simulink library "smartTruckLib"  (R2018b)
settings: Solver=VariableStepAuto  StartTime=0.0  StopTime=10.0  RelTol=1e-3
values from neighbouring files (symbols this model uses):
  actorDest = 0    [modelParams.m]
  initYPos = 0    [modelParams.m]
  laneWidth = laneSpecification.Width    [modelParams.m]
  minOverlapJourney = 200    [modelParams.m]
  platoonFuelSavings = 20    [modelParams.m]
  safeTimeGap = 1.4    [modelParams.m]
  standStillGap = 10    [modelParams.m]
undefined symbols (not defined in the file or in its folder): DiscIntNeverNeededParam, key, setActorTableEntry, tableEntry
libraries: mpcadaslib x1
settings Model: Creator=surongal  LastModifiedBy=surongal
settings DataIOCC: ReturnWorkspaceOutputs=on

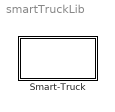
== system smartTruckLib ==
  Smart-Truck : Subsystem  InitFcn=|  mask(Truck){initXPos=100, destXPos=5000, initXVel=10, maxAcceleration=3, maxDeceleration=-6, maxVelocity=30, truckId=1}
      | % To get the offset for the truckId
      | numTrucks = actorCount();
      | truckXPosition(numTrucks) = str2num( get_param(gcb,'initXPos'));
      | truckVelocity(numTrucks) = str2num( get_param(gcb,'initXVel'));
      | % To set the truckId
      | set_param(gcb,'truckId',num2str(numTrucks + truckIdBase));
      | destXPos = get_param(gcb,'destXPos');
      | actorDest(truckIdBase + numTrucks) = str2num(destXPos);
      mask prompts: initXPos "Initial X-position"; destXPos "Destination X-Position"; initXVel "Initial X-velocity"; maxAcceleration "Max acceleration"; maxDeceleration "Max deceleration"; maxVelocity "Max velocity"; truckId "id"
      mask help: This block allows to introduce a smart-truck in the scenario.
      mask Display: image('icons/truck.png');

== system smartTruckLib/Smart-Truck ==
  note: Smart Truck
  Actor-system : Subsystem
  Bus Selector : BusSelector  OutputSignals=ActorID
  Load Initial Pose : MATLAB Function  TreatAsAtomicUnit=on
  Publish to Table : FunctionCaller  FunctionPrototype=setActorTableEntry(key,tableEntry)
  wires:
  Load Initial Pose/1(initTruckPose) -> Actor-system/1(Initial Truck Pose)
  Actor-system/1(Updated Pose) -> Publish to Table/2, Bus Selector/1
  Bus Selector/1 -> Publish to Table/1  "<ActorID>"

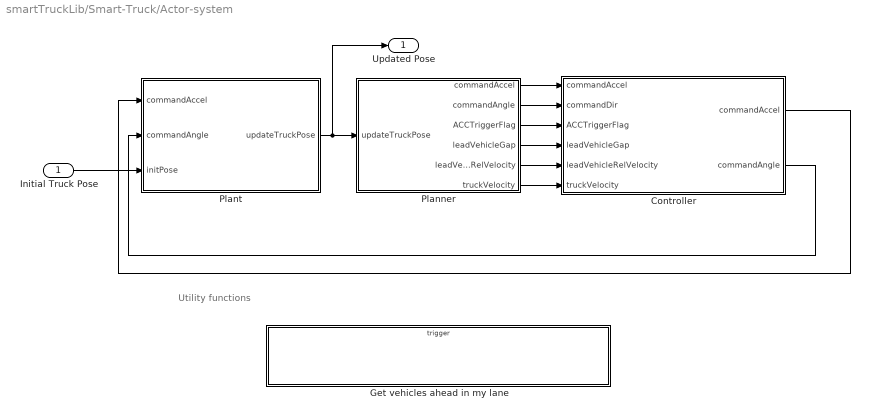
== system smartTruckLib/Smart-Truck/Actor-system ==
  note: Utility functions
  Initial Truck Pose : Inport
  Controller : Subsystem
  Get vehicles ahead in my lane : Subsystem  TreatAsAtomicUnit=on
  Planner : Subsystem
  Plant : Subsystem
  Updated Pose : Outport
  wires:
  Planner/6(truckVelocity) -> Controller/6(" truckVelocity")
  Planner/5(leadVehicleRelVelocity) -> Controller/5(" leadVehicleRelVelocity")
  Planner/4(leadVehicleGap) -> Controller/4(" leadVehicleGap")
  Planner/3(ACCTriggerFlag) -> Controller/3(ACCTriggerFlag)
  Planner/2(commandAngle) -> Controller/2(" commandDir")
  Planner/1(commandAccel) -> Controller/1(" commandAccel")
  Plant/1(updateTruckPose) -> Updated Pose/1, Planner/1(updateTruckPose)
  Controller/1(commandAccel) -> Plant/1(" commandAccel")
  Initial Truck Pose/1 -> Plant/3(initPose)
  Controller/2(commandAngle) -> Plant/2(commandAngle)

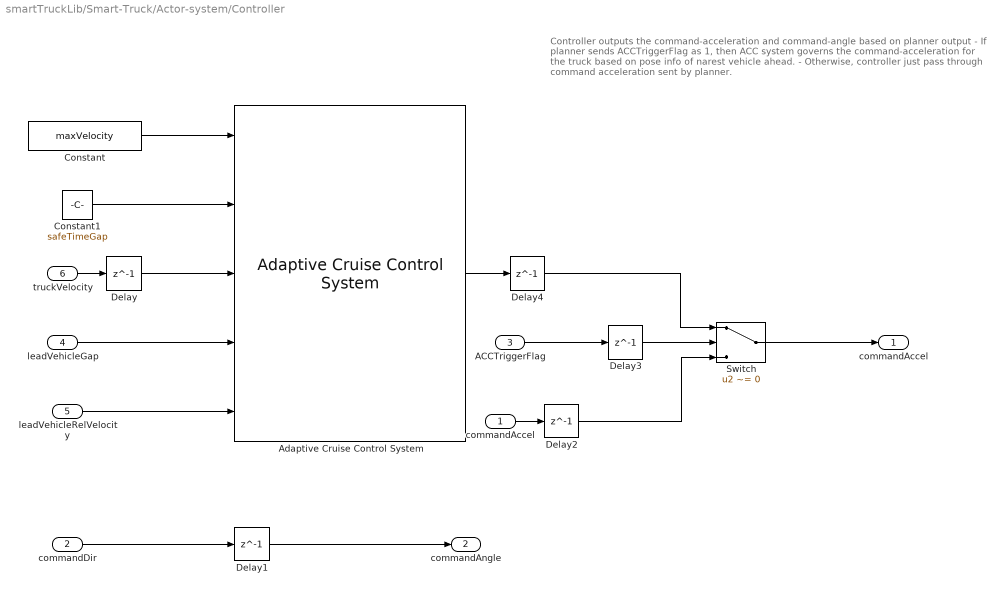
== system smartTruckLib/Smart-Truck/Actor-system/Controller ==
  note: Controller outputs the command-acceleration and command-angle
      | based on planner output
      | - If planner sends ACCTriggerFlag as 1, then ACC system governs the
      |   command-acceleration for the truck based on pose info
      |   of narest vehicle ahead.
      | - Otherwise, controller just pass through command acceleration
      |   sent by planner.
  " commandAccel" : Inport
  " commandDir" : Inport  Port=2
  ACCTriggerFlag : Inport  Port=3
  " leadVehicleGap" : Inport  Port=4
  " leadVehicleRelVelocity" : Inport  Port=5
  " truckVelocity" : Inport  Port=6
  Adaptive Cruise Control System : mpcadaslib/Adaptive Cruise Control System  EgoModel=tf(1,[0.5,1,0])  InitialEgoVelocity=abs(initXVel)  DefaultSpacing=standStillGap  MaxVelocity=maxVelocity  MinAcceleration=maxDeceleration  amin_ext=off  MaxAcceleration=maxAcceleration  amax_ext=off  Ts=0.1  PredictionHorizon=30  ControllerBehavior=0.5  suboptimal=off  maxiter=10  datatypeopt=double  optmode=off  trackmode=off
      settings: SourceProductName=Model Predictive Control Toolbox
  Constant : Constant  Value=maxVelocity  SampleTime=-1
  Constant1 : Constant  Value=safeTimeGap
  Delay{,1..4} (5 alike) : Delay  DelayLength=1  InitialCondition=0
  Switch : Switch  Criteria=u2 ~= 0
  commandAccel : Outport
  commandAngle : Outport  Port=2
  wires:
  Constant1/1 -> Adaptive Cruise Control System/2
  Adaptive Cruise Control System/1 -> Delay4/1
  Delay4/1 -> Switch/1
  Delay3/1 -> Switch/2
  Delay2/1 -> Switch/3
  Switch/1 -> commandAccel/1
  ACCTriggerFlag/1 -> Delay3/1
  " truckVelocity"/1 -> Delay/1
  Delay1/1 -> commandAngle/1
  Delay/1 -> Adaptive Cruise Control System/3
  " commandDir"/1 -> Delay1/1
  " leadVehicleRelVelocity"/1 -> Adaptive Cruise Control System/5
  " leadVehicleGap"/1 -> Adaptive Cruise Control System/4
  Constant/1 -> Adaptive Cruise Control System/1
  " commandAccel"/1 -> Delay2/1

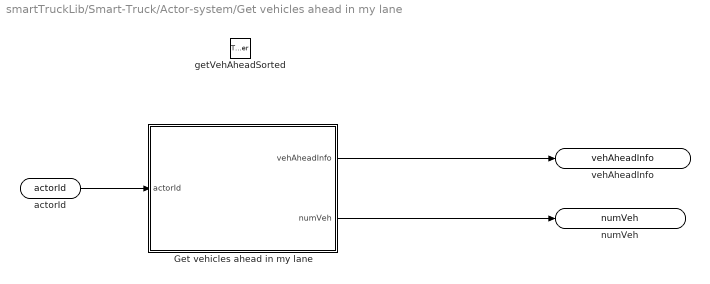
== system smartTruckLib/Smart-Truck/Actor-system/Get vehicles ahead in my lane ==
  getVehAheadSorted : TriggerPort  TriggerType=function-call  IsSimulinkFunction=on  FunctionName=getVehAheadSorted  FunctionVisibility=scoped  VariantControl=(inherit)
  Get vehicles ahead in my lane : MATLAB Function  TreatAsAtomicUnit=on
  actorId : ArgIn  ArgumentName=actorId
  numVeh : ArgOut  ArgumentName=numVeh
  vehAheadInfo : ArgOut  Port=2  OutDataTypeStr=Bus: Vehicle  PortDimensions=maxVehicles  ArgumentName=vehAheadInfo
  wires:
  Get vehicles ahead in my lane/2(numVeh) -> numVeh/1
  Get vehicles ahead in my lane/1(vehAheadInfo) -> vehAheadInfo/1
  actorId/1 -> Get vehicles ahead in my lane/1(actorId)

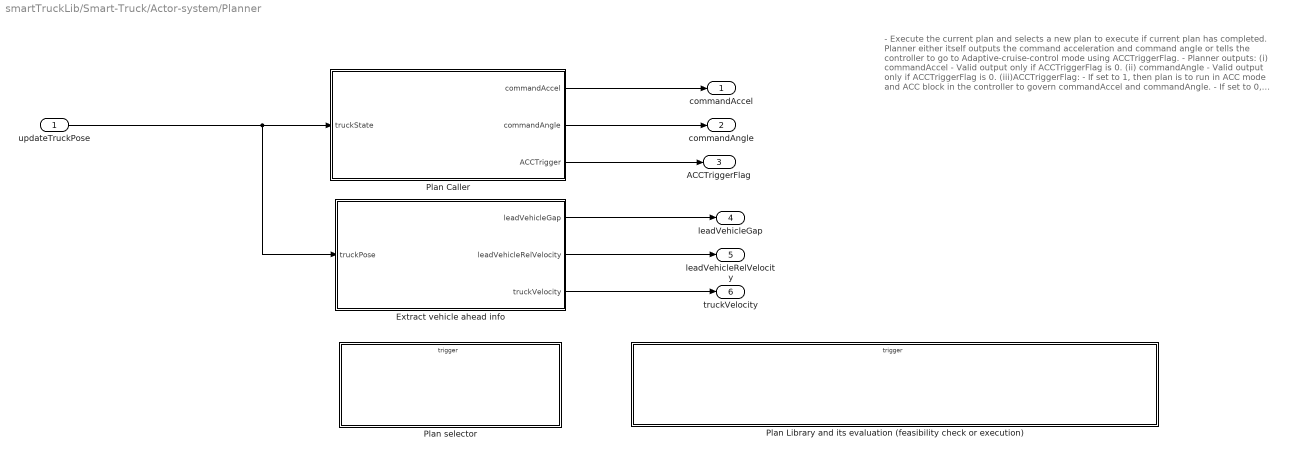
== system smartTruckLib/Smart-Truck/Actor-system/Planner ==
  note: - Execute the current plan and selects a new plan to execute if
      | current plan has completed. Planner either itself outputs the command
      | acceleration and command angle or tells the controller to go to
      | Adaptive-cruise-control mode using ACCTriggerFlag.
      |
      | - Planner outputs:
      | (i) commandAccel -  Valid output only if ACCTriggerFlag is 0.
      | (ii) commandAngle - Valid output only if ACCTriggerFlag is 0.
      | (iii)ACCTriggerFlag:
      |        - If set to 1, then plan is to run in ACC mode and ACC
      |          block in the controller to govern commandAccel and
      |          commandAngle.
      |        - If set to 0, then planner itself gives the commandAccel and
      |          commandAngle.
      | (iv) Other 3 outputs (leadVehicleGap, leadVehicleVelocity, truckVelocity)
      |       are the required inputs for ACC controlled movement and controller
      |       uses them only if ACCTriggerFlag = 1
  updateTruckPose : Inport
  Extract vehicle ahead info : MATLAB Function  TreatAsAtomicUnit=on
  Plan Caller : MATLAB Function  TreatAsAtomicUnit=on
  "Plan Library and its evaluation (feasibility check or execution) " : Subsystem  TreatAsAtomicUnit=on
  Plan selector : Subsystem  TreatAsAtomicUnit=on
  commandAccel : Outport
  commandAngle : Outport  Port=2
  ACCTriggerFlag : Outport  Port=3
  leadVehicleGap : Outport  Port=4
  leadVehicleRelVelocity : Outport  Port=5
  truckVelocity : Outport  Port=6
  wires:
  Plan Caller/3(ACCTrigger) -> ACCTriggerFlag/1
  Extract vehicle ahead info/3(truckVelocity) -> truckVelocity/1
  Extract vehicle ahead info/1(leadVehicleGap) -> leadVehicleGap/1
  Extract vehicle ahead info/2(leadVehicleRelVelocity) -> leadVehicleRelVelocity/1
  Plan Caller/2(commandAngle) -> commandAngle/1
  Plan Caller/1(commandAccel) -> commandAccel/1
  updateTruckPose/1 -> Plan Caller/1(truckState), Extract vehicle ahead info/1(truckPose)

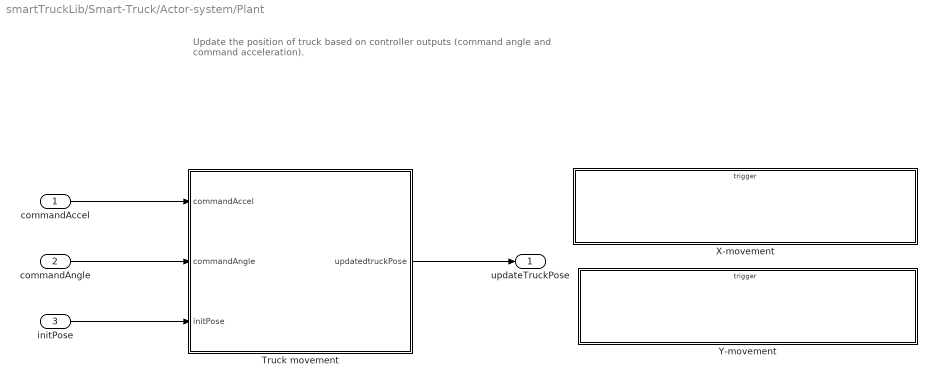
== system smartTruckLib/Smart-Truck/Actor-system/Plant ==
  note: Update the position of truck based on controller outputs
      |  (command angle and command acceleration).
  " commandAccel" : Inport
  commandAngle : Inport  Port=2
  initPose : Inport  Port=3
  Truck movement : MATLAB Function  TreatAsAtomicUnit=on
  X-movement : Subsystem  TreatAsAtomicUnit=on
  Y-movement : Subsystem  TreatAsAtomicUnit=on
  updateTruckPose : Outport
  wires:
  commandAngle/1 -> Truck movement/2(commandAngle)
  " commandAccel"/1 -> Truck movement/1(commandAccel)
  Truck movement/1(updatedtruckPose) -> updateTruckPose/1
  initPose/1 -> Truck movement/3(initPose)

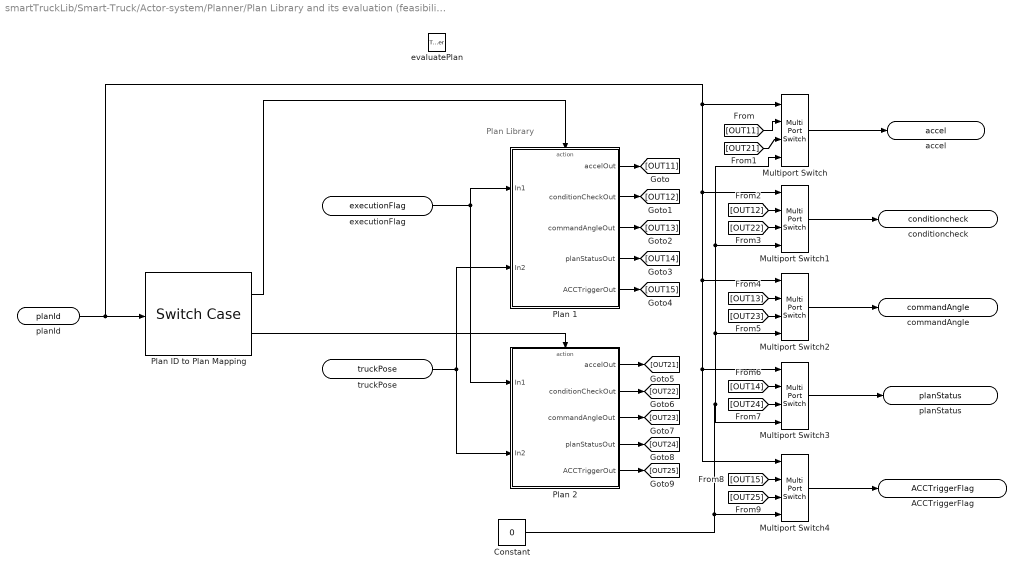
== system smartTruckLib/Smart-Truck/Actor-system/Planner/Plan Library and its evaluation (feasibility check or execution)  ==
  note: Plan Library
  evaluatePlan : TriggerPort  TriggerType=function-call  IsSimulinkFunction=on  FunctionName=evaluatePlan  FunctionVisibility=scoped  VariantControl=(inherit)
  Constant : Constant  Value=0  SampleTime=-1
  Multiport Switch{,1..4} (5 alike) : MultiPortSwitch  Inputs=2  DataPortForDefault=Additional data port
  Plan 1 : Subsystem  TreatAsAtomicUnit=on
  Plan 2 : Subsystem  TreatAsAtomicUnit=on
  Plan ID to Plan Mapping : SwitchCase  CaseConditions={1,2}  ShowDefaultCase=off
  planId : ArgIn  DisableCoverage=on  ArgumentName=planId
  executionFlag : ArgIn  Port=2  ArgumentName=executionFlag
  truckPose : ArgIn  Port=3  OutDataTypeStr=Bus: Vehicle  ArgumentName=truckPose
  accel : ArgOut  DisableCoverage=on  ArgumentName=accel
  conditioncheck : ArgOut  DisableCoverage=on  Port=2  ArgumentName=conditioncheck
  commandAngle : ArgOut  DisableCoverage=on  Port=3  ArgumentName=commandAngle
  planStatus : ArgOut  DisableCoverage=on  Port=4  ArgumentName=planStatus
  ACCTriggerFlag : ArgOut  DisableCoverage=on  Port=5  ArgumentName=ACCTriggerFlag
  wires:
  Multiport Switch4/1 -> ACCTriggerFlag/1
  Multiport Switch3/1 -> planStatus/1
  Multiport Switch1/1 -> conditioncheck/1
  Multiport Switch2/1 -> commandAngle/1
  Multiport Switch/1 -> accel/1
  truckPose/1 -> Plan 1/2(In2), Plan 2/2(In2)
  executionFlag/1 -> Plan 1/1(In1), Plan 2/1(In1)
  Plan ID to Plan Mapping/1 -> Plan 1/Action
  Plan ID to Plan Mapping/2 -> Plan 2/Action
  [OUT22] -> Multiport Switch1/3
  [OUT24] -> Multiport Switch3/3
  [OUT11] -> Multiport Switch/2
  [OUT21] -> Multiport Switch/3
  [OUT12] -> Multiport Switch1/2
  [OUT15] -> Multiport Switch4/2
  [OUT13] -> Multiport Switch2/2
  [OUT23] -> Multiport Switch2/3
  [OUT14] -> Multiport Switch3/2
  Constant/1 -> Multiport Switch1/4, Multiport Switch/4, Multiport Switch2/4, Multiport Switch3/4, Multiport Switch4/4
  planId/1 -> Multiport Switch1/1, Multiport Switch2/1, Multiport Switch4/1, Multiport Switch3/1, Multiport Switch/1, Plan ID to Plan Mapping/1
  [OUT25] -> Multiport Switch4/3
  Plan 1/1(accelOut) -> [OUT11]
  Plan 1/2(conditionCheckOut) -> [OUT12]
  Plan 1/3(commandAngleOut) -> [OUT13]
  Plan 1/4(planStatusOut) -> [OUT14]
  Plan 1/5(ACCTriggerOut) -> [OUT15]
  Plan 2/5(ACCTriggerOut) -> [OUT25]
  Plan 2/4(planStatusOut) -> [OUT24]
  Plan 2/3(commandAngleOut) -> [OUT23]
  Plan 2/2(conditionCheckOut) -> [OUT22]
  Plan 2/1(accelOut) -> [OUT21]

== system smartTruckLib/Smart-Truck/Actor-system/Planner/Plan selector ==
  selectNewPlan : TriggerPort  TriggerType=function-call  IsSimulinkFunction=on  FunctionName=selectNewPlan  FunctionVisibility=scoped  VariantControl=(inherit)
  Choose plan : MATLAB Function  TreatAsAtomicUnit=on
  truckPose : ArgIn  OutDataTypeStr=Bus: Vehicle  ArgumentName=truckPose
  planID : ArgOut  DisableCoverage=on  ArgumentName=planID
  wires:
  truckPose/1 -> Choose plan/1(truckPose)
  Choose plan/1(planId) -> planID/1

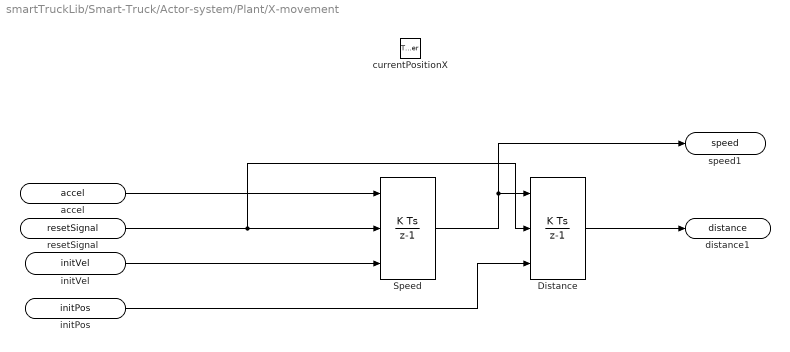
== system smartTruckLib/Smart-Truck/Actor-system/Plant/X-movement ==
  currentPositionX : TriggerPort  TriggerType=function-call  IsSimulinkFunction=on  FunctionName=currentPositionX  FunctionVisibility=scoped  VariantControl=(inherit)
  Distance : DiscreteIntegrator  ExternalReset=level  InitialConditionSource=external  SampleTime=-1  ICPrevOutput=DiscIntNeverNeededParam  ICPrevScaledInput=DiscIntNeverNeededParam
  Speed : DiscreteIntegrator  ExternalReset=level  InitialConditionSource=external  SampleTime=-1  LimitOutput=on  LowerSaturationLimit=0  ICPrevOutput=DiscIntNeverNeededParam  ICPrevScaledInput=DiscIntNeverNeededParam
  accel : ArgIn  ArgumentName=accel
  resetSignal : ArgIn  Port=2  ArgumentName=resetSignal
  initVel : ArgIn  Port=3  ArgumentName=initVel
  initPos : ArgIn  Port=4  ArgumentName=initPos
  distance1 : ArgOut  ArgumentName=distance
  speed1 : ArgOut  Port=2  ArgumentName=speed
  wires:
  initVel/1 -> Speed/3
  resetSignal/1 -> Speed/2, Distance/2
  accel/1 -> Speed/1
  Distance/1 -> distance1/1
  Speed/1 -> speed1/1, Distance/1
  initPos/1 -> Distance/3

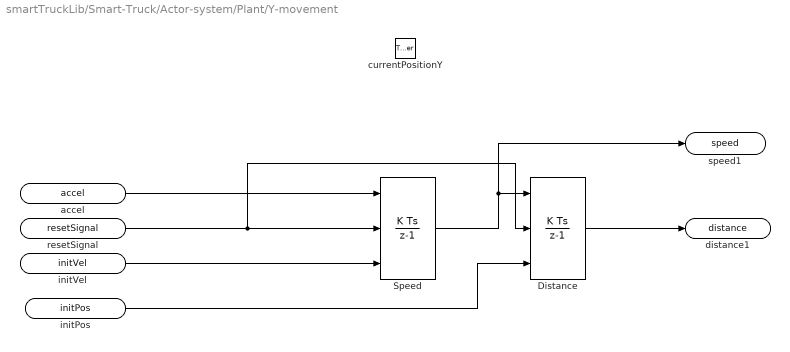
== system smartTruckLib/Smart-Truck/Actor-system/Plant/Y-movement ==
  currentPositionY : TriggerPort  TriggerType=function-call  IsSimulinkFunction=on  FunctionName=currentPositionY  FunctionVisibility=scoped  VariantControl=(inherit)
  Distance : DiscreteIntegrator  ExternalReset=level  InitialConditionSource=external  SampleTime=-1  ICPrevOutput=DiscIntNeverNeededParam  ICPrevScaledInput=DiscIntNeverNeededParam
  Speed : DiscreteIntegrator  ExternalReset=level  InitialConditionSource=external  SampleTime=-1  LimitOutput=on  LowerSaturationLimit=0  ICPrevOutput=DiscIntNeverNeededParam  ICPrevScaledInput=DiscIntNeverNeededParam
  accel : ArgIn  ArgumentName=accel
  resetSignal : ArgIn  Port=2  ArgumentName=resetSignal
  initVel : ArgIn  Port=3  ArgumentName=initVel
  initPos : ArgIn  Port=4  ArgumentName=initPos
  distance1 : ArgOut  ArgumentName=distance
  speed1 : ArgOut  Port=2  ArgumentName=speed
  wires:
  resetSignal/1 -> Speed/2, Distance/2
  accel/1 -> Speed/1
  Speed/1 -> speed1/1, Distance/1
  Distance/1 -> distance1/1
  initPos/1 -> Distance/3
  initVel/1 -> Speed/3

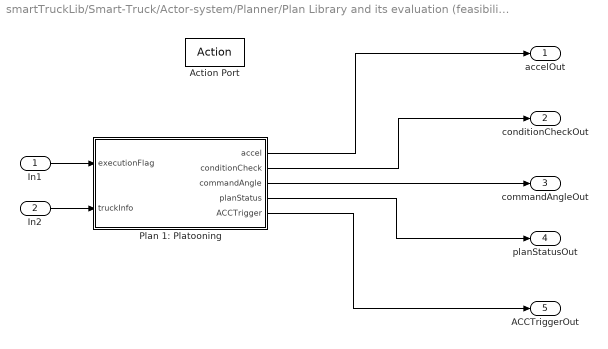
== system smartTruckLib/Smart-Truck/Actor-system/Planner/Plan Library and its evaluation (feasibility check or execution) /Plan 1 ==
  In1 : Inport
  In2 : Inport  Port=2  OutDataTypeStr=Bus: Vehicle
  Action Port : ActionPort
  Plan 1: Platooning : Stateflow chart  TreatAsAtomicUnit=on
  accelOut : Outport
  conditionCheckOut : Outport  Port=2
  commandAngleOut : Outport  Port=3
  planStatusOut : Outport  Port=4
  ACCTriggerOut : Outport  Port=5
  wires:
  Plan 1: Platooning/4(planStatus) -> planStatusOut/1
  Plan 1: Platooning/5(ACCTrigger) -> ACCTriggerOut/1
  Plan 1: Platooning/2(conditionCheck) -> conditionCheckOut/1
  Plan 1: Platooning/3(commandAngle) -> commandAngleOut/1
  Plan 1: Platooning/1(accel) -> accelOut/1
  In1/1 -> Plan 1: Platooning/1(executionFlag)
  In2/1 -> Plan 1: Platooning/2(truckInfo)

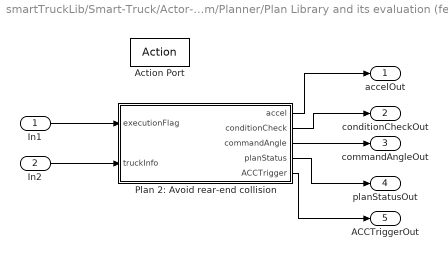
== system smartTruckLib/Smart-Truck/Actor-system/Planner/Plan Library and its evaluation (feasibility check or execution) /Plan 2 ==
  In1 : Inport
  In2 : Inport  Port=2
  Action Port : ActionPort
  Plan 2: Avoid rear-end collision : Stateflow chart  TreatAsAtomicUnit=on
  accelOut : Outport
  conditionCheckOut : Outport  Port=2
  commandAngleOut : Outport  Port=3
  planStatusOut : Outport  Port=4
  ACCTriggerOut : Outport  Port=5
  wires:
  Plan 2: Avoid rear-end collision/5(ACCTrigger) -> ACCTriggerOut/1
  Plan 2: Avoid rear-end collision/4(planStatus) -> planStatusOut/1
  Plan 2: Avoid rear-end collision/2(conditionCheck) -> conditionCheckOut/1
  Plan 2: Avoid rear-end collision/3(commandAngle) -> commandAngleOut/1
  Plan 2: Avoid rear-end collision/1(accel) -> accelOut/1
  In2/1 -> Plan 2: Avoid rear-end collision/2(truckInfo)
  In1/1 -> Plan 2: Avoid rear-end collision/1(executionFlag)

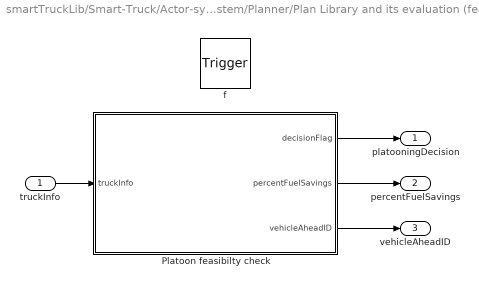
== system smartTruckLib/Smart-Truck/Actor-system/Planner/Plan Library and its evaluation (feasibility check or execution) /Plan 1/Plan 1: Platooning/checkPlatoonFeasibility ==
  truckInfo : Inport  OutDataTypeStr=Bus: Vehicle  PortDimensions=1
  f : TriggerPort  TriggerType=function-call  VariantControl=(inherit)
      settings: CopyFcn=Stateflow.SLINSF.SimulinkMan.removeBlockPreDeleteFcn  PreDeleteFcn=Stateflow.SLINSF.SimulinkMan.unsafePredeleteFcn
  Platoon feasibilty check : Stateflow chart  TreatAsAtomicUnit=on
  platooningDecision : Outport
  percentFuelSavings : Outport  Port=2
  vehicleAheadID : Outport  Port=3
  wires:
  truckInfo/1 -> Platoon feasibilty check/1(truckInfo)
  Platoon feasibilty check/1(decisionFlag) -> platooningDecision/1
  Platoon feasibilty check/2(percentFuelSavings) -> percentFuelSavings/1
  Platoon feasibilty check/3(vehicleAheadID) -> vehicleAheadID/1

== stateflow chart smartTruckLib/Smart-Truck/Actor-system/Planner/Plan Library and its evaluation (feasibility check or execution) /Plan 1/Plan 1: Platooning/checkPlatoonFeasibility/Platoon feasibilty check ==
  state Check whether forming a platoon is possible and it is beneficial to do so in terms of fuel savings. [group]
    - Fuel savings during the platoon comes from the fact, that a truck folowing another one experiences much reduced aerodynamic drag
    and typically saves (15-20 %) fuel.
    - Fuel consumtions also depends on the velocity and acceleration of truck.
    Combing the factors affecting the fuel consumption, it is anticipated whether it could be beneficial to form platoon with truck ahead.
    - Decision Flag represents one of the following condition
    decisionFlag = 1 : Platooning is anticipated to give better fuel efficiency
    decisionFlag = 2 : Platoon not formed as truck has reached the destination
    decisionFlag = 3 : No truck ahead to form platoon with
    decisionFlag = 4 : Platoon not formed as truck cannot match up to the velocity of truck ahead
    decisionFlag = 5 : Platoon not formed due to small overlapping journey
    decisionFlag = 6 : Platoon not formed as the truck cannot cover the excess gap
    decisionFlag = 7 : Platooning is anticipated to be more fuel consuming
    decisionFlag = 8 : Platoon not formed as one of the truck is anticipated to reach the destination before forming the platoon
  (default) -> (junction 145) : {
      |    decisionFlag = 0;
      |    percentFuelSavings = 0;
      |    [numVeh vehiclesAheadInfo] = getVehAheadSorted(truckInfo.ActorID);
      |    i=1;
      | }
  (junction 145) -> (junction 141) [order 1] : [i<=numVeh]
  (junction 140) -> (junction 145) : {
      |      i=i+1;
      | }
  (junction 145) -> (junction 156) [order 2]
  (junction 141) -> (junction 140) : {
      |     % Convert to self-centered pose
      |      vehiclesAheadInfo(i) = ...
      |      globalToEgoCentered(truckInfo, vehiclesAheadInfo(i));
      | }
  (junction 156) -> (junction 1) [order 1] : [truckInfo.Position(1) < actorDest(truckInfo.ActorID)]
  (junction 1) -> (junction 4) [order 1] : % If there is a truck ahead
      |         [numVeh > 0]
  (junction 156) -> (junction 161) [order 2] : {
      |   decisionFlag = 2;
      | }
  (junction 1) -> (junction 93) [order 2] : {
      |    decisionFlag = 3;
      | }
  (junction 4) -> (junction 89) : {
      |     nearestVeh = vehiclesAheadInfo(1);   % Details of nearest vehicle ahead
      |     nearestVehDest = actorDest(nearestVeh.ActorID);
      |     truckDest = actorDest(truckInfo.ActorID);
      |     nearestVehAbsVel = truckInfo.Velocity(1) + nearestVeh.Velocity(1); % Absolute Speed of Vehicle ahead
      |
      | }
  (junction 89) -> (junction 93) [order 2] : % Platooning not feasible
      | {
      |    decisionFlag = 4;
      | }
  (junction 89) -> (junction 91) [order 1] : % Platooning is not possible if this
      | % truck cannot match up to the
      | % velocity of truck ahead.
      | [nearestVehAbsVel <= maxVelocity]
  (junction 93) -> (junction 55)
  (junction 91) -> (junction 6) : {
      |     nearestVehAbsPos = truckInfo.Position(1) + nearestVeh.Position(1); % Absolute Position of Vehicle ahead
      |     % overlapping journey end point of two actors.
      |     overlapEndpoint = min( truckDest, nearestVehDest);
      |     % overlap journey distance of two vehicles
      |     overlapDistance = overlapEndpoint - (nearestVehAbsPos);
      | }
  (junction 6) -> (junction 55) [order 2] : % Platooning not feasible
      | {
      |    decisionFlag = 5;
      | }
  (junction 6) -> (junction 8) [order 1] : % If overlapping journey is bigger than the
      | % minimum required for platooning
      | [overlapDistance >= minOverlapJourney]
  (junction 8) -> (junction 32) : {
      |     dToOverlapEP = overlapEndpoint - truckInfo.Position(1); % distance to overlap end point
      |     % Estimated time required to reach overlap end point with zero acceleration
      |     tToDest = dToOverlapEP/truckInfo.Velocity(1);
      |     % Anticipated fuel consumption if truck keeps moving with its current speed
      |     % without going for platooning.
      |     fuelNoPlatoon = fuelConsumptionCalculator(truckInfo.Velocity(1),0,tToDest);
      |     excessGap = nearestVeh.Position(1) - ((safeTimeGap * (nearestVehAbsVel)) ...
      |               + standStillGap); % gap iin addition to required safe Gap
      | }
  (junction 55) -> (junction 114)
  (junction 107) -> (junction 114) [order 1] : % Can't cover the excessGap vehicle ahead is moving at higher speed
      | [maxVelocity < ...
      |  nearestVehAbsVel+1]
      | {
      |  decisionFlag = 6;
      | }
  (junction 34) -> (junction 107) [order 1] : [excessGap>0]
  (junction 32) -> (junction 34) [order 1] : % If vehicle ahead is moving at higher speed
      |             [nearestVeh.Velocity(1) > 0]
  (junction 107) -> (junction 120) [order 2] : {
      | % Accelerate to become faster
      |  % than veh ahead (by 1m/s)
      | ta1 = (nearestVeh.Velocity(1)+1)/ ...
      |        maxAcceleration;
      | fa1 = fuelConsumptionCalculator( ...
      |         truckInfo.Velocity(1), ...
      |         maxAcceleration,ta1);
      | d1 = (truckInfo.Velocity(1)* ta1)+ ...
      |    ((0.5)*maxAcceleration* (ta1^2));
      | remGap = excessGap - d1 + ...
      |    (nearestVehAbsVel*ta1) ;
      | }
  (junction 34) -> (junction 36) [order 2] : {
      |    % No excess gap, only need to match
      |    % the speed up
      |    ta = (nearestVeh.Velocity(1))/maxAcceleration;
      |    % Distance travelled to form the platoon
      |    dToFormPlatoon = (truckInfo.Velocity(1)* ta)+ ...
      |    ((0.5)*maxAcceleration* (ta^2));
      |    % fuel to form platoon
      |    fa = fuelConsumptionCalculator( ...
      |          truckInfo.Velocity(1),maxAcceleration,ta);
      | }
  (junction 32) -> (junction 97) [order 2]
  (junction 114) -> (junction 44)
  (junction 97) -> (junction 98) [order 1] : [excessGap > 0]
      | % If Excess Gap to be covered
  (junction 97) -> (junction 37) [order 2] : {
      |     dToFormPlatoon = 0;
      |     fa = 0;
      | }
  (junction 98) -> (junction 101) : {
      |    % Applying relative motion
      |    u = -nearestVeh.Velocity(1);
      |
      |    %time required to form the platoon
      |    ta =  (-u + sqrt((u^2) + 2* maxAcceleration* excessGap))/ ...
      |            maxAcceleration;
      |    % Distance travelled to form the platoon
      |    dToFormPlatoon = (truckInfo.Velocity(1)* ta)+((0.5)*maxAcceleration* (ta^2));
      |    % fuel to form platoon
      |    fa = fuelConsumptionCalculator( ...
      |          truckInfo.Velocity(1),maxAcceleration,ta);
      |
      | }
  (junction 120) -> (junction 122) [order 1] : [remGap < 0]
  (junction 120) -> (junction 124) [order 2] : {
      | % Cover the pending excess gap
      | ta2  = remGap/1;
      | fa2 =fuelConsumptionCalculator( ...
      |         nearestVehAbsVel+1, ...
      |         0,ta2);
      | d2 = (nearestVehAbsVel+1) ...
      |         *ta2;
      | % Distance travelled to form the
      | % platoon
      | dToFormPlatoon = d1 + d2;
      | % Anticipated fuel consumption to
      | % form platoon
      | fa = fa1 + fa2;
      | }
  (junction 122) -> (junction 117) : {
      | dToFormPlatoon ...
      |  = d1;
      | fa = fa1;
      | }
  (junction 124) -> (junction 117)
  (junction 117) -> (junction 36)
  (junction 37) -> (junction 36)
  (junction 101) -> (junction 37)
  (junction 36) -> (junction 42)
  (junction 42) -> (junction 44) [order 1] : % If overlapping journey end point is going to be overshot
      | % by this truck vehicle before forming the platoon itself,
      | % then decide against forming the platoon.
      | [(truckInfo.Position(1) + dToFormPlatoon) > overlapEndpoint]
      | {
      |     decisionFlag = 8;
      | }
  (junction 44) -> (junction 49)
  (junction 42) -> (junction 47) [order 2] : {
      |         journeyInPlatoon = ((overlapEndpoint - truckInfo.Position(1)) - dToFormPlatoon);
      |         % Time after formation of platoon upto end of overlapping journey  i.e. journey time as part of platoon
      |         tb = (journeyInPlatoon) / (nearestVehAbsVel);
      |         % Anticipated fuel consumption when truck is moving as part of
      |         % platoon. Fuel savings due to platooning are also applied
      |         fb = ((100-platoonFuelSavings)/100)*fuelConsumptionCalculator(nearestVehAbsVel,0,tb);
      |
      |         % Total anticipated fuel consumption with platooning
      |         fuelPlatoon = fa + fb;
      | }
  (junction 47) -> (junction 49) [order 1] : % Platoon is not fuel effecient
      | [fuelPlatoon > fuelNoPlatoon]
      | {
      |     decisionFlag = 7;
      | }
  (junction 49) -> (junction 60)
  (junction 47) -> (junction 53) [order 2] : {
      |     % Fuel efficient
      |     decisionFlag = 1;
      |     percentFuelSavings = (fuelNoPlatoon - fuelPlatoon)*(100/fuelPlatoon);
      |     vehicleAheadID = vehiclesAheadInfo(1).ActorID;
      | }
  (junction 60) -> (junction 161)
  (junction 53) -> (junction 60)
  data: speed function_input; accel function_input; time function_input; fuelConsumption function_output; truckInfo input Bus: Vehicle; nearestVehDest local; nearestVeh local Bus: Vehicle; numVeh local; overlapDistance local; overlapEndpoint local; vehiclesAheadInfo local Bus: Vehicle; minOverlapJourney parameter; truckDest local; actorDest parameter; maxAcceleration parameter; platoonFuelSavings parameter; safeTimeGap parameter; standStillGap parameter; decisionFlag output; dToFormPlatoon local; dToOverlapEP local; fuelNoPlatoon local; fuelPlatoon local; journeyInPlatoon local; nearestVehAbsPos local; nearestVehAbsVel local; ta local; tb local; u local; fa local; fb local; tToDest local; maxVelocity parameter; excessGap local; percentFuelSavings output; d1 local; d2 local; fa1 local; fa2 local; remGap local; ta1 local; ta2 local; vehicleAheadID output; i local
  function fuelConsumption = fuelConsumptionCalculator(speed,accel,time):
    | function fuelConsumption = fuelConsumptionCalculator(speed,accel,time)
    | % fuel consumption model
    | b = [0.1569, 0.02450,-0.0007415,0.00005975];
    | c = [0.07224, 0.09681,0.001075];
    | fuelConsumption = time * (accel * (c(1) + c(2)*speed + c(3)*speed^2) +(b(1) + b(2)*speed + b(3)*speed^2 + b(4)*speed^3));
    | end

== stateflow chart smartTruckLib/Smart-Truck/Actor-system/Planner/Plan Library and its evaluation (feasibility check or execution) /Plan 1/Plan 1: Platooning ==
  settings: executeAtInitialization=1
  state [platooningDecision, percentFuelSavings, vehicleAheadID] = checkPlatoonFeasibility(truckInfo) [function]
  state Platooning Plan: [group]
    - Truck forms platoon with the actor ahead. This arrangement continues till one of them reaches its destination.
    - Although a truck forms a platoon with the truck ahead only if it anticipates platooning to be fuel-saving.
  state MoveAsPlatoon
    entry:
    platoonJourneyCompleted = 0;
    [numVehAhead vehiclesAheadInfo] = getVehAheadSorted(truckInfo.ActorID);
    for i=1:numVehAhead % Convert to self-centered pose
    vehiclesAheadInfo(i) = globalToEgoCentered(truckInfo, vehiclesAheadInfo(i));
    end
    nearestVeh = vehiclesAheadInfo(1);   % Nearest vehicle Ahead
    nearestVehDest = actorDest(nearestVeh.ActorID);
    truckDest = actorDest(truckInfo.ActorID);
    nearestVehAbsPos = truckInfo.Position(1) + nearestVeh.Position(1); % Absolute Position of Vehicle ahead
    % overlapping journey end point of two actors.
    overlapEndpoint = min( truckDest, nearestVehDest);
    commandAngle = 0;
    accel = 0;
    ACCTrigger = 1;
    during:
    [numVehAhead vehiclesAheadInfo] = getVehAheadSorted(truckInfo.ActorID);
    for i=1:numVehAhead % Convert to self-centered pose
    vehiclesAheadInfo(i) = globalToEgoCentered(truckInfo, vehiclesAheadInfo(i));
    end
    % Truck reached destination
    if(truckInfo.Position(1)  >= overlapEndpoint)
    % This marks completion of journey of truck as platoon
    platoonJourneyCompleted = 1;
    end
    exit:
    percentFuelSavings = 0;
    planStatus = 0;
    truckPlatoonInfo.PlatoonStatus = 0;
    truckPlatoonInfo.FuelSavings = percentFuelSavings;
    truckPlatoonInfo.VehicleAheadID = 0;
    setVisualizationTableEntry(truckPlatoonInfo.ActorID, truckPlatoonInfo); % Write into visualization data-table.
  state FeasibilityCheckofPlatoon
    entry:
    conditionCheck = 0;
    ACCTrigger = 0;
    percentFuelSavings = 0;
    during:
    [conditionCheck percentFuelSavings, vehicleAheadID] = checkPlatoonFeasibility(truckInfo);
    truckPlatoonInfo.ActorID = truckInfo.ActorID;
    if conditionCheck == 1
    truckPlatoonInfo.PlatoonStatus = 1;
    truckPlatoonInfo.FuelSavings = percentFuelSavings;
    truckPlatoonInfo.VehicleAheadID = vehicleAheadID;
    else
    truckPlatoonInfo.PlatoonStatus = conditionCheck;
    truckPlatoonInfo.FuelSavings = percentFuelSavings;
    truckPlatoonInfo.VehicleAheadID = 0;
    end
    setVisualizationTableEntry(truckPlatoonInfo.ActorID, truckPlatoonInfo); % Write into visualization data-table
  (default) -> FeasibilityCheckofPlatoon
  MoveAsPlatoon -> FeasibilityCheckofPlatoon : [platoonJourneyCompleted == 1  || ...
      |  numVehAhead == 0]
  FeasibilityCheckofPlatoon -> MoveAsPlatoon : [conditionCheck==1 && executionFlag ==1]
      | % Move as platoon and follow the truck ahead
  data: truckInfo function_input Bus: Vehicle size=1; platooningDecision function_output; percentFuelSavings function_output; vehicleAheadID function_output; executionFlag input; accel output; conditionCheck output; commandAngle output; planStatus output; ACCTrigger output; truckInfo input Bus: Vehicle; actorDest parameter; nearestVehAbsPos local; nearestVeh local Bus: Vehicle; nearestVehDest local; overlapEndpoint local; platoonJourneyCompleted local; vehiclesAheadInfo local Bus: Vehicle; numVehAhead local; percentFuelSavings local; truckPlatoonInfo local Bus: PlatoonStatistics; vehicleAheadID local; i local; truckDest local

== matlab function smartTruckLib/Smart-Truck/Load Initial Pose ==
  data: initTruckPose output Bus: Vehicle; truckId parameter; initXPos parameter; initYPos parameter; initXVel parameter
function initTruckPose = loadTruckInitPose(truckId, initXPos, initYPos, initXVel)
% Write initial pose entry into the actor pose table and return the same

persistent truckPose;
if(isempty(truckPose))
    truckPose = struct('ActorID', truckId, 'Position', [initXPos initYPos 0], ...
        'Velocity', [abs(initXVel) 0 0], 'Roll', 0, 'Pitch', 0, 'Yaw', 0, ...
        'AngularVelocity', [0 0 0]);
    setActorTableEntry(truckId, truckPose);
end
initTruckPose = truckPose;

== matlab function smartTruckLib/Smart-Truck/Actor-system/Get vehicles ahead in my lane/Get vehicles ahead in my lane ==
  data: actorId input; vehAheadInfo output Bus: Vehicle size=maxVehicles; numVeh output; maxVehicles parameter
function [vehAheadInfo, numVeh]  = getVehAheadSorted(actorId, maxVehicles)
% Call the data-table query for getting the list of vehicles ahead
% and returns the sorted list of those vehicles in increasing order of
% their distance from truck.
actorStruct = struct('ActorID', 0, 'Position', [0 0 0], ...
    'Velocity', [0 0 0], 'Roll', 0, 'Pitch', 0, 'Yaw', 0, ...
    'AngularVelocity', [0 0 0]);
vehAheadInfo = repmat(actorStruct, maxVehicles, 1);
qHdl = initActorQueryIterator(actorId, uint32(PlatooningQueries.VehiclesAhead));
[key, done] = getActorQueryIterNextKey(qHdl);
mIdx = 1;
% Get next vehicle-of-interest and insert in a sorted way in order of its
% distance from truck.
while ~done
    info = getActorTableEntry(key);
    if(mIdx == 1) % First vehicle
        vehAheadInfo(mIdx) = info;
    else
        i= (mIdx - 1);
        while(i >= 1 && (info.Position(1) < vehAheadInfo(i).Position(1))) %Insert at correct place to maintain sorted order
            vehAheadInfo(i + 1) = vehAheadInfo(i);
            i = i - 1;
        end
        vehAheadInfo(i + 1) = info;
    end
    mIdx = mIdx + 1;
    [key, done] = getActorQueryIterNextKey(qHdl);
end
numVeh = mIdx - 1;

== matlab function smartTruckLib/Smart-Truck/Actor-system/Planner/Extract vehicle ahead info ==
  data: leadVehicleGap output; leadVehicleRelVelocity output; truckPose input; maxVelocity parameter; truckVelocity output; safeTimeGap parameter; standStillGap parameter
function [leadVehicleGap, leadVehicleRelVelocity, truckVelocity] = getVehAheadInfo( ...
    truckPose, maxVelocity, safeTimeGap, standStillGap)
% Get Lead vehicle info for Adaptive cruise control mode.

truckVelocity = truckPose.Velocity(1);
[numVeh, vehAheadInfo] = getVehAheadSorted(truckPose.ActorID);
for i = 1 : numVeh % Convert to self-centered pose
    vehAheadInfo(i) = globalToEgoCentered(truckPose, vehAheadInfo(i));
end
if(numVeh > 0) % If there is a vehicle ahead
    leadVehicleGap = vehAheadInfo(1).Position(1);
    leadVehicleRelVelocity = vehAheadInfo(1).Velocity(1);
else
    % Set to max sensing range to give an impression that there is no
    % vehicle ahead and hence ego-car can go full throttle.
    leadVehicleGap = safeTimeGap * maxVelocity + standStillGap;
    leadVehicleRelVelocity = 0;
end

== matlab function smartTruckLib/Smart-Truck/Actor-system/Planner/Plan Caller ==
  data: truckState input; commandAccel output; commandAngle output; ACCTrigger output
function [commandAccel, commandAngle, ACCTrigger]  = planSelectAndExecute(truckState)
% Execute the current plan and select a new plan to execute if cureent plan
% has completed.

persistent planId;
persistent planStatus;
commandAngle = 0;
commandAccel = 0;
ACCTrigger = 0;
if isempty(planStatus)
    % no plan is selected
    planId = 0;
    planStatus = 0;
end
if(planStatus == 0) % If no plan is runnning/some plan has completed
    planId = selectNewPlan(truckState);
end
if(planId > 0) % Execute the plan (either newly selected or ongoing)
    [commandAccel, ~, commandAngle, planStatus, ACCTrigger] = evaluatePlan(planId, 1, truckState);
else
     planStatus = 0;
end

== stateflow chart smartTruckLib/Smart-Truck/Actor-system/Planner/Plan Library and its evaluation (feasibility check or execution) /Plan 2/Plan 2: Avoid rear-end collision ==
  settings: executeAtInitialization=1
  state Plan to avoid collision with vehicle ahead . [group]
    - If there is a vehicle ahead, decelerate if required to maintain the safe gap.
    - Otherwise accelerate to reach optimal velocity for maximum fuel effeciency.
  (default) -> (junction 158) : {
      | conditionCheck = 0;
      | }
  (junction 158) -> (junction 232) [order 1] : [truckInfo.Position(1) < actorDest(truckInfo.ActorID)]
      |           % Not yet reached destination
  (junction 158) -> (junction 159) [order 2]
  (junction 232) -> (junction 230) : {
      |     conditionCheck = 1;
      | }
  (junction 230) -> (junction 159) [order 2]
  (junction 230) -> (junction 150) [order 1] : % Whether to execute plan
      | [executionFlag == 1]
  (junction 159) -> (junction 156)
  (junction 150) -> (junction 253) : {
      |       accel = 0;
      |       commandAngle = 0;
      |       ACCTrigger = 0;
      |       % Get vehicles ahead
      |       [numVeh vehiclesAheadInfo] = getVehAheadSorted(truckInfo.ActorID);
      |       i=1;
      | }
  (junction 253) -> (junction 250) [order 1] : [i<=numVeh]
  (junction 257) -> (junction 253) : {
      | i=i+1;
      | }
  (junction 253) -> (junction 154) [order 2]
  (junction 250) -> (junction 257) : {
      |     % Convert to self-centered pose
      |      vehiclesAheadInfo(i) = ...
      |      globalToEgoCentered(truckInfo, vehiclesAheadInfo(i));
      | }
  (junction 154) -> (junction 155) [order 1] : % If there is a vehicle ahead and it has not yet reached its destination
      | [numVeh > 0  && ((vehiclesAheadInfo(1).Position(1) + truckInfo.Position(1) ) < actorDest(vehiclesAheadInfo(1).ActorID)) ]
  (junction 154) -> (junction 217) [order 3]
  (junction 154) -> (junction 181) [order 2] : [truckInfo.Velocity(1) < initXVel]
  (junction 155) -> (junction 212) : {
      |     % Accelerate/Decelerate if required
      |     accel = checkForAcceleration(truckInfo.Velocity(1), ....
      |            vehiclesAheadInfo(1).Position(1));
      | }
  (junction 181) -> (junction 184) : {
      |     % Accelerate to achieve max. fuel effeciency
      |     accel =  maxAcceleration
      | }
  (junction 217) -> (junction 156) : {
      |      planStatus = 0;
      | }
  (junction 184) -> (junction 217)
  (junction 212) -> (junction 184)
  data: truckVel function_input; gap function_input; safeTimeGap parameter; maxDeceleration parameter; acceleration function_output; standStillGap parameter; accel output; executionFlag input; conditionCheck output; commandAngle output; truckInfo input Bus: Vehicle; vehiclesAheadInfo local Bus: Vehicle; numVeh local; maxAcceleration parameter; planStatus output; ACCTrigger output; actorDest parameter; initXVel parameter; i local
  function acceleration = checkForAcceleration(truckVel, gap):
    | function acceleration = checkForAcceleration(truckVel, gap)
    | % Calculate required deceleration to maintain safe gap
    | % If gap is more than safe-gap  required, then check if there is any
    | % acceleration required to reach desired velocity (i.e. initial velocity)
    | acceleration = 0;
    | additionalSafeGap = 10; % Vehicle to accelerate only if it has additional
    | % precautionary safety gap on top of required safe-gap.
    | safeGap = (truckVel * safeTimeGap) + standStillGap;
    | if(gap < safeGap)
    |     acceleration = maxDeceleration ;
    | elseif(gap > ((safeGap + additionalSafeGap)) && (truckVel < initXVel))
    |     acceleration = maxAcceleration;
    | end

== matlab function smartTruckLib/Smart-Truck/Actor-system/Planner/Plan selector/Choose plan ==
  data: planId output; truckPose input; numPlans parameter
function planId = findFeasiblePlan( truckPose, numPlans)
% Find a plan which has highest priority and is feasible based on entry
% condition

planId = 0;
executionFlag = 0; % Only feasibility of plan is checked, plan is not executed
% Loop through all the plans to select one
for index = 1 : numPlans
    [~, conditionCheck, ~, ~] = evaluatePlan(index, executionFlag, truckPose);
    if(conditionCheck == 1)
        planId = index;
        return;
    end
end

== matlab function smartTruckLib/Smart-Truck/Actor-system/Plant/Truck movement ==
  data: commandAccel input; commandAngle input; initPose input; updatedtruckPose output Bus: Vehicle; actorDest parameter; laneWidth parameter
function updatedtruckPose  = simulateTruckMovement(commandAccel, commandAngle, initPose, actorDest, laneWidth)
% Update the position of truck based on controller outputs (command
% angle and command acceleration)

persistent truckPose;
persistent prevCommandAngle;
persistent initVelocityX;
persistent initPositionX;
persistent initVelocityY;
persistent initPositionY;
persistent vehStopFlag;
if isempty(truckPose)
    truckPose = initPose;
    prevCommandAngle = 0;
    initVelocityX = initPose.Velocity(1);
    initPositionX = initPose.Position(1);
    initVelocityY = initPose.Velocity(2);
    initPositionY = initPose.Position(2);
end

if(truckPose.Position(1) >= actorDest(truckPose.ActorID)) % Check to make sure that truck stops at destination.
    if(isempty(vehStopFlag))
        truckPose.Velocity(1) = 0;
        truckPose.Position(2) = truckPose.Position(2) + (laneWidth/2 + 2); % Move it aside
        vehStopFlag = 1;
    end
else
    speed =  sqrt(truckPose.Velocity(1) * truckPose.Velocity(1) + truckPose.Velocity(2) * truckPose.Velocity(2));
    if truckPose.Velocity(1) <= 0 && commandAccel < 0 % To avoid backward movement
        commandAccel = 0;
        truckPose.Velocity(1) = 0;
        [truckPose.Position(1), truckPose.Velocity(1)] = currentPositionX(...
            commandAccel * cosd(commandAngle), 1, truckPose.Velocity(1), truckPose.Position(1)); % For x-dir
        [truckPose.Position(2), truckPose.Velocity(2)] = currentPositionY(...
            commandAccel * sind(commandAngle), 1, truckPose.Velocity(2), truckPose.Position(2)); % For y-dir
        initPositionX = truckPose.Position(1);
        initPositionY = truckPose.Position(2);
        initVelocityX = truckPose.Velocity(1);
        initVelocityY = truckPose.Velocity(2);
    else
        if(commandAngle == prevCommandAngle )
            [truckPose.Position(1), truckPose.Velocity(1)] = currentPositionX(commandAccel * cosd(commandAngle), ...
                0, initVelocityX, initPositionX ); % For x-dir
            [truckPose.Position(2), truckPose.Velocity(2)] = currentPositionY(commandAccel * sind(commandAngle), ...
                0, initVelocityY, initPositionY); % For y-dir
        else
            % When direction changes, reset the two integrator blocks and set current value as initial value.
            initVelocityX = speed * cosd(commandAngle);
            initVelocityY = speed * sind(commandAngle);
            [truckPose.Position(1), truckPose.Velocity(1)] = currentPositionX(commandAccel * cosd(commandAngle), ...
                1, initVelocityX, truckPose.Position(1) ); % For x-dir
            [truckPose.Position(2), truckPose.Velocity(2)] = currentPositionY(commandAccel * sind(commandAngle),...
                1, initVelocityY, truckPose.Position(2)); % For y-dir
            initPositionX = truckPose.Position(1);
            initPositionY = truckPose.Position(2);
        end
    end
end
prevCommandAngle = commandAngle;
updatedtruckPose = truckPose;
